simulink model "FinproPMSMSensor"  (R2021b)
settings: Solver=VariableStepAuto  StartTime=0.0  StopTime=10  FixedStep=1e-6  RelTol=1e-3
settings Model: Creator=skadi  LastModifiedBy=skadi

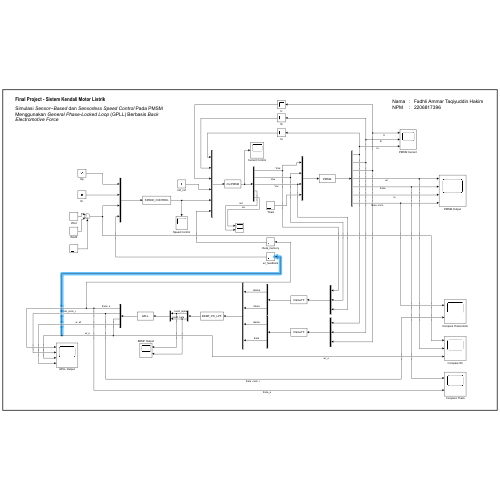
[thumbnail: Simulink's stored preview of the top-level diagram]
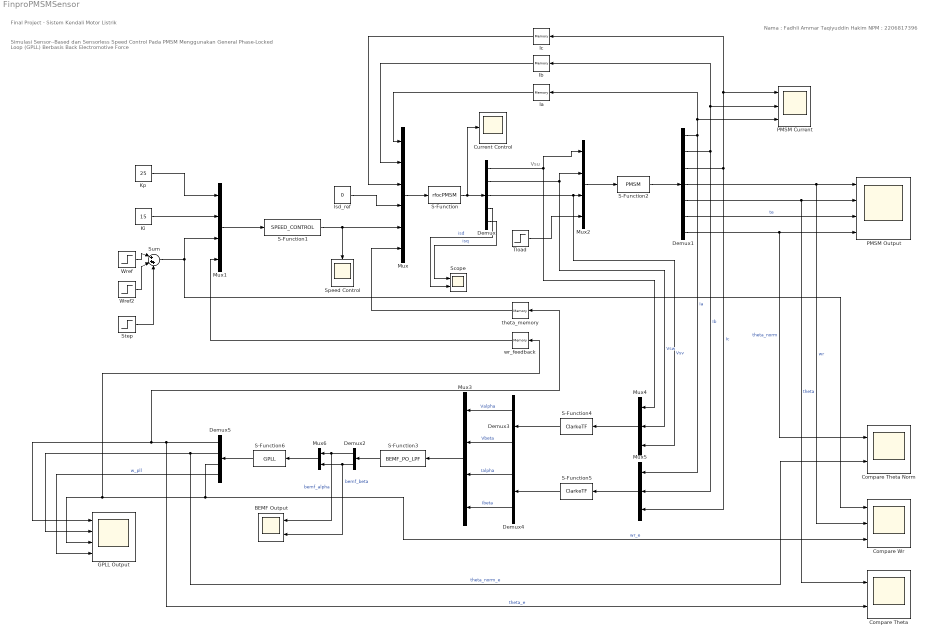
== system FinproPMSMSensor ==
  note: Nama : Fadhli Ammar Taqiyuddin Hakim
      | NPM : 2206817396
  note: Final Project - Sistem Kendali Motor Listrik
  note: Vsu
  note: Simulasi Sensor--Based dan Sensorless Speed Control Pada PMSM Menggunakan General Phase-Locked Loop (GPLL) Berbasis Back Electromotive Force
  BEMF Output : Scope  NumInputPorts=2
  Compare Theta : Scope  NumInputPorts=2
  Compare Theta Norm : Scope  NumInputPorts=2
  Compare Wr : Scope  NumInputPorts=3
  Current Control : Scope
  Demux : Demux  Outputs=5
  Demux1 : Demux  Outputs=7
  Demux2 : Demux  Outputs=2
  Demux3 : Demux  Outputs=2
  Demux4 : Demux  Outputs=2
  Demux5 : Demux
  GPLL Output : Scope  NumInputPorts=4
  Ia : Memory
  Ib : Memory
  Ic : Memory
  Isd_ref : Constant  Value=0
  Ki : Constant  Value=15
  Kp : Constant  Value=25
  Mux : Mux  Inputs=6
  Mux1 : Mux
  Mux2 : Mux
  Mux3 : Mux
  Mux4 : Mux  Inputs=3
  Mux5 : Mux  Inputs=3
  Mux6 : Mux  Inputs=2
  PMSM Current : Scope  NumInputPorts=3
  PMSM Output : Scope  NumInputPorts=4
  S-Function : S-Function  FunctionName=rfocPMSM  SFunctionDeploymentMode=off  EnableBusSupport=off
  S-Function1 : S-Function  FunctionName=SPEED_CONTROL  SFunctionDeploymentMode=off  EnableBusSupport=off
  S-Function2 : S-Function  FunctionName=PMSM  SFunctionDeploymentMode=off  EnableBusSupport=off
  S-Function3 : S-Function  FunctionName=BEMF_PO_LPF  SFunctionDeploymentMode=off  EnableBusSupport=off
  S-Function4 : S-Function  FunctionName=ClarkeTF  SFunctionDeploymentMode=off  EnableBusSupport=off
  S-Function5 : S-Function  FunctionName=ClarkeTF  SFunctionDeploymentMode=off  EnableBusSupport=off
  S-Function6 : S-Function  FunctionName=GPLL  SFunctionDeploymentMode=off  EnableBusSupport=off
  Scope : Scope  NumInputPorts=2
  Speed Control : Scope
  Step : Step  Time=5  After=100  SampleTime=0
  Sum : Sum  Inputs=|+++
  Tload : Step  Time=5  After=0  SampleTime=0
  Wref : Step  After=50  SampleTime=0
  Wref2 : Step  Time=3  After=-100  SampleTime=0
  theta_memory : Memory
  wr_feedback : Memory
  wires:
  Demux/3 -> Mux4/3, Mux2/3  "Vsv"
  Demux/1 -> Mux2/1, Mux4/1
  Mux2/1 -> S-Function2/1
  Tload/1 -> Mux2/4
  Demux/2 -> Mux4/2, Mux2/2  "Vsw"
  S-Function/1 -> Current Control/1, Demux/1
  Mux/1 -> S-Function/1
  S-Function2/1 -> Demux1/1
  S-Function1/1 -> Mux/5, Speed Control/1
  Demux1/1 -> Mux5/1, PMSM Current/3, Ia/1  "Ia"
  Ia/1 -> Mux/1
  Ib/1 -> Mux/2
  Ic/1 -> Mux/3
  Demux1/2 -> Mux5/2, Ib/1, PMSM Current/2  "Ib"
  Demux1/3 -> Mux5/3, Ic/1, PMSM Current/1  "Ic"
  Demux1/4 -> Compare Wr/2, PMSM Output/1  "wr"
  Demux1/5 -> Compare Theta/1, PMSM Output/2  "theta"
  Demux1/6 -> PMSM Output/3  "te"
  Mux1/1 -> S-Function1/1
  theta_memory/1 -> Mux/6
  wr_feedback/1 -> Mux1/4
  Kp/1 -> Mux1/1
  Ki/1 -> Mux1/2
  Isd_ref/1 -> Mux/4
  Demux1/7 -> Compare Theta Norm/1, PMSM Output/4  "theta_norm"
  Mux3/1 -> S-Function3/1
  S-Function3/1 -> Demux2/1
  Mux4/1 -> S-Function4/1
  S-Function4/1 -> Demux3/1
  Demux3/1 -> Mux3/1  "Valpha"
  Demux3/2 -> Mux3/2  "Vbeta"
  S-Function5/1 -> Demux4/1
  Mux5/1 -> S-Function5/1
  Demux4/1 -> Mux3/3  "Ialpha"
  Demux4/2 -> Mux3/4  "Ibeta"
  S-Function6/1 -> Demux5/1
  Mux6/1 -> S-Function6/1
  Demux2/1 -> BEMF Output/1, Mux6/1  "bemf_alpha"
  Demux2/2 -> BEMF Output/2, Mux6/2  "bemf_beta"
  Demux5/2 -> Compare Theta Norm/2, GPLL Output/2  "theta_norm_e"
  Demux5/3 -> Compare Wr/3, wr_feedback/1, GPLL Output/3  "wr_e"
  Demux5/1 -> Compare Theta/2, theta_memory/1, GPLL Output/1  "theta_e"
  Demux5/4 -> GPLL Output/4  "w_pll"
  Demux/4 -> Scope/2  "isd"
  Demux/5 -> Scope/1  "isq"
  Wref/1 -> Sum/1
  Sum/1 -> Compare Wr/1, Mux1/3
  Wref2/1 -> Sum/2
  Step/1 -> Sum/3
